simulink model "mbd_projecet"  (R2023b)
settings: Solver=VariableStepAuto  StartTime=0.0  StopTime=10.0  RelTol=1e-3
settings Model: Creator=Ahmed  LastModifiedBy=Ahmed

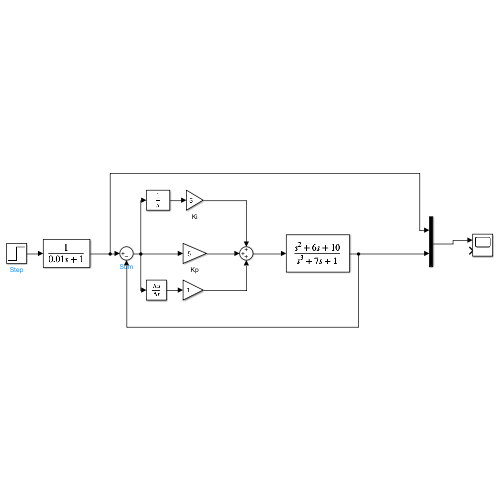
[thumbnail: Simulink's stored preview of the top-level diagram]
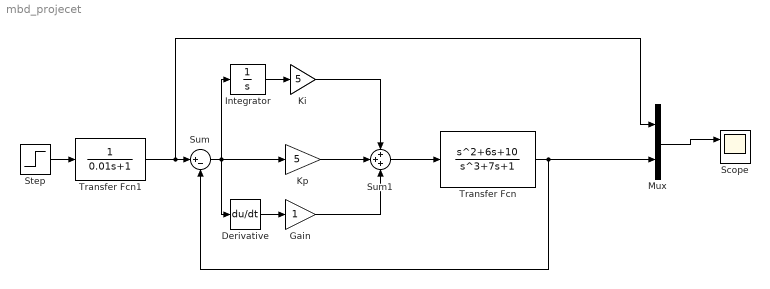
== system mbd_projecet ==
  Derivative : Derivative
  Gain : Gain
  Integrator : Integrator
  Ki : Gain  Gain=5
  Kp : Gain  Gain=5
  Mux : Mux  Inputs=2
  Scope : Scope  NumInputPorts=2
  Step : Step  SampleTime=0
  Sum : Sum  Inputs=|+-
  Sum1 : Sum  Inputs=+++
  Transfer Fcn : TransferFcn  Numerator=[1,6,10]  Denominator=[1,0,7,1]
  Transfer Fcn1 : TransferFcn  Denominator=[0.01,1]
  wires:
  Sum/1 -> Derivative/1, Integrator/1, Kp/1
  Step/1 -> Transfer Fcn1/1
  Transfer Fcn/1 -> Mux/2, Sum/2
  Mux/1 -> Scope/1
  Integrator/1 -> Ki/1
  Derivative/1 -> Gain/1
  Ki/1 -> Sum1/1
  Kp/1 -> Sum1/2
  Gain/1 -> Sum1/3
  Sum1/1 -> Transfer Fcn/1
  Transfer Fcn1/1 -> Mux/1, Sum/1
